simulink library "airlib"  (Simulink 8.7)
settings: Solver=VariableStepAuto  SolverMode=SingleTasking  StartTime=0.0  StopTime=10.0  RelTol=1e-3
undefined symbols (not defined in the file or in its folder): DiscIntNeverNeededParam
libraries: airlib x2
(part 2 of 2)

== system airlib/DT-B747/ad/ad3 ==
  x : Inport
  yatm : Inport  Port=2
  yad1 : Inport  Port=3
  0 : Subsystem
      mask Display: disp('AIRDATA3\nM.O. Rauw, October 1997')
  Mux : Mux  Inputs=3
  Mux1 : Mux  Inputs=[12 5 3]
  Re : Fcn  Expr=(u[13]*u[1])/u[16]
  Tt : Fcn  Expr=u[15] * (1+0.2*u[19]^2)
  cbar : Gain  Gain=cbar  SaturateOnIntegerOverflow=on  OutDataTypeStr=Inherit: Same as input  ParamDataTypeStr=Inherit: Same as input
  yad3 : Outport
  wires:
  yad1/1 -> Mux1/3
  yatm/1 -> Mux1/2
  x/1 -> Mux1/1
  Re/1 -> Mux/2, cbar/1
  Mux1/1 -> Re/1, Tt/1
  Mux/1 -> yad3/1
  Tt/1 -> Mux/1
  cbar/1 -> Mux/3

== system airlib/DT-B747/ad/atm ==
  x : Inport
  0 : Subsystem
      mask Display: disp('ATMOSPH\nM.O. Rauw, October 1997')
  Mux : Mux  Inputs=2
  Mux1 : Mux  Inputs=[2 1]
  Mux2 : Mux  Inputs=5
  T : Fcn  Expr=288.15 - 0.0065*u[12]
  g : Fcn  Expr=9.80665*(6371020/(6371020+u[12]))^2
  mu : Fcn  Expr=(1.458*10^(-6)*u[2]^1.5)/(u[2]+110.4)
  ps : Fcn  Expr=101325*(u[2]/288.15)^(u[1]/1.86584)
  rho : Fcn  Expr=u[3]/(287.053*u[2])
  yatm : Outport
  wires:
  x/1 -> T/1, g/1
  Mux/1 -> Mux1/1, mu/1, ps/1
  ps/1 -> Mux1/2, Mux2/2
  T/1 -> Mux/2, Mux2/3
  g/1 -> Mux/1, Mux2/5
  rho/1 -> Mux2/1
  Mux1/1 -> rho/1
  Mux2/1 -> yatm/1
  mu/1 -> Mux2/4

== system airlib/DT-B747/ae/0 ==

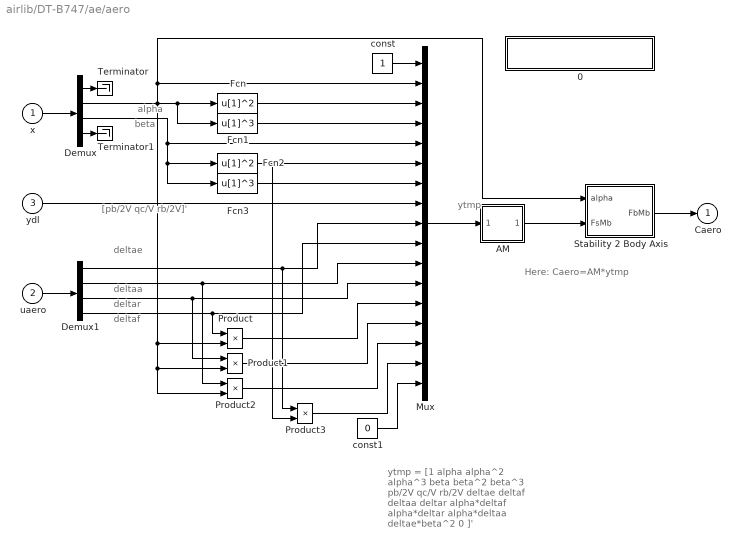
== system airlib/DT-B747/ae/aero ==
  note: ytmp = [1  alpha  alpha^2  alpha^3  beta  beta^2  beta^3  pb/2V  qc/V  rb/2V  deltae
      | deltaf  deltaa  deltar  alpha*deltaf  alpha*deltar  alpha*deltaa  deltae*beta^2  0 ]'
  note: [pb/2V qc/V rb/2V]'
  note: beta
  note: deltae
  note: deltaa
  note: deltar
  note: deltaf
  note: alpha
  note: ytmp
  note: Here: Caero=AM*ytmp
  x : Inport
  uaero : Inport  Port=2
  ydl : Inport  Port=3
  0 : Subsystem
      mask Display: disp('AEROMOD\nM.O. Rauw, October 1997')
  "AM " : Subsystem  mask(State Space){M=AM}
      mask prompts: M "Matrix"
      mask Display: disp('Matrix\nGain')
  Demux : Demux  Outputs=[1 1 1 9]
  Demux1 : Demux
  Fcn : Fcn  Expr=u[1]^2
  Fcn1 : Fcn  Expr=u[1]^3
  Fcn2 : Fcn  Expr=u[1]^2
  Fcn3 : Fcn  Expr=u[1]^3
  Mux : Mux  Inputs=[1 1 1 1 1 1 1 3 1 1 1 1 1 1 1 1 1]
  Product{,1..3} (4 alike) : Product  SaturateOnIntegerOverflow=on  RndMeth=Zero  InputSameDT=on  OutDataTypeStr=Inherit: Same as first input
  Stability 2 Body Axis : Subsystem
  Terminator : Terminator
  Terminator1 : Terminator
  const : Constant
  const1 : Constant  Value=0
  Caero : Outport
  wires:
  Demux/4 -> Terminator1/1
  Demux/1 -> Terminator/1
  const1/1 -> Mux/17
  const/1 -> Mux/1
  ydl/1 -> Mux/8
  Product3/1 -> Mux/16
  Product2/1 -> Mux/15
  Product1/1 -> Mux/14
  Demux1/1 -> Mux/9, Product3/1
  Fcn2/1 -> Mux/6, Product3/2
  Demux1/4 -> Mux/10, Product/1
  Demux/2 -> Fcn/1, Fcn1/1, Product/2, Product1/2, Product2/2, Mux/2, Stability 2 Body Axis/1(alpha)
  Demux/3 -> Mux/5, Fcn2/1, Fcn3/1
  Demux1/2 -> Mux/11, Product2/1
  Demux1/3 -> Mux/12, Product1/1
  Product/1 -> Mux/13
  Fcn3/1 -> Mux/7
  uaero/1 -> Demux1/1
  Fcn1/1 -> Mux/4
  Fcn/1 -> Mux/3
  x/1 -> Demux/1
  Mux/1 -> "AM "/1(In1)
  Stability 2 Body Axis/1(FbMb) -> Caero/1
  "AM "/1(Out1) -> Stability 2 Body Axis/2(FsMb)

== system airlib/DT-B747/ae/dl ==
  x : Inport
  0 : Subsystem
      mask Display: disp('DIMLESS\nM.O. Rauw, October 1997')
  Mux : Mux  Inputs=3
  pb/2V : Fcn  Expr=0.5 * u[4] * b / u[1]
  qc/2V : Fcn  Expr=0.5* u[5] * cbar / u[1]
  rb/2V : Fcn  Expr=0.5 * u[6] * b / u[1]
  ydl : Outport
  wires:
  pb/2V/1 -> Mux/1
  qc/2V/1 -> Mux/2
  rb/2V/1 -> Mux/3
  Mux/1 -> ydl/1
  x/1 -> qc/2V/1, rb/2V/1, pb/2V/1

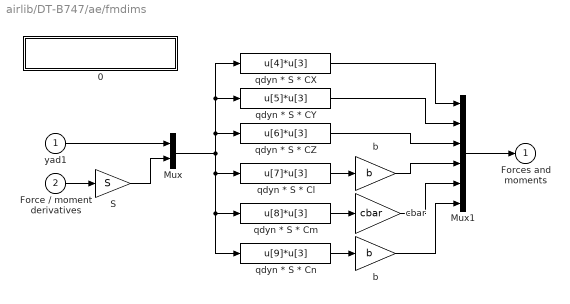
== system airlib/DT-B747/ae/fmdims ==
  yad1 : Inport
  Force / moment derivatives : Inport  Port=2
  0 : Subsystem
      mask Display: disp('FMDIMS\nM.O. Rauw, October 1997')
  Mux : Mux  Inputs=[3 6]
  Mux1 : Mux  Inputs=6
  S : Gain  Gain=S  SaturateOnIntegerOverflow=on  OutDataTypeStr=Inherit: Same as input  ParamDataTypeStr=Inherit: Same as input
  b : Gain  Gain=b  SaturateOnIntegerOverflow=on  OutDataTypeStr=Inherit: Same as input  ParamDataTypeStr=Inherit: Same as input
  "b " : Gain  Gain=b  SaturateOnIntegerOverflow=on  OutDataTypeStr=Inherit: Same as input  ParamDataTypeStr=Inherit: Same as input
  cbar : Gain  Gain=cbar  SaturateOnIntegerOverflow=on  OutDataTypeStr=Inherit: Same as input  ParamDataTypeStr=Inherit: Same as input
  qdyn * S * CX : Fcn  Expr=u[4]*u[3]
  qdyn * S * CY : Fcn  Expr=u[5]*u[3]
  qdyn * S * CZ : Fcn  Expr=u[6]*u[3]
  qdyn * S * Cl : Fcn  Expr=u[7]*u[3]
  qdyn * S * Cm : Fcn  Expr=u[8]*u[3]
  qdyn * S * Cn : Fcn  Expr=u[9]*u[3]
  Forces and moments : Outport
  wires:
  Mux1/1 -> Forces and moments/1
  "b "/1 -> Mux1/6
  cbar/1 -> Mux1/5
  Force / moment derivatives/1 -> S/1
  Mux/1 -> qdyn * S * CZ/1, qdyn * S * CX/1, qdyn * S * CY/1, qdyn * S * Cl/1, qdyn * S * Cm/1, qdyn * S * Cn/1
  qdyn * S * Cl/1 -> b/1
  qdyn * S * Cm/1 -> cbar/1
  qdyn * S * Cn/1 -> "b "/1
  yad1/1 -> Mux/1
  qdyn * S * CX/1 -> Mux1/1
  qdyn * S * CY/1 -> Mux1/2
  S/1 -> Mux/2
  qdyn * S * CZ/1 -> Mux1/3
  b/1 -> Mux1/4

== system airlib/DT-B747/eqm/0 ==

== system airlib/DT-B747/eqm/? ==

== system airlib/DT-B747/eqm/ODE ==
  x : Inport
  Ftot : Inport  Port=2
  Mtot : Inport  Port=3
  yhlp : Inport  Port=4
  ybvel* : Inport  Port=5
  0 : Subsystem
      mask Display: disp('12 Ordinary Differential\nEquations (level 4)\nM.O. Rauw')
  Eulerdot : Subsystem  mask(Eulerdot){}
      mask help:
      | Calculation of d(psi)/dt, d(theta)/dt,
      | and d(phi/dt)
      mask Display: disp('psi dot\ntheta dot\nphi dot')
  Mux : Mux  Inputs=[12 3 3 11]
  Mux1 : Mux  Inputs=[3 3 3 3]
  Vabdot : Subsystem  mask(Vabdot){m=GM1(10)}
      mask prompts: m "Mass of the aircraft [kg]:"
      mask help: Calculation of dV/dt, dalpha/dt, dbeta/dt.
      mask Display: disp('V dot\nalpha dot\nbeta dot')
  pqrdot : Subsystem  mask(pqrdot){}
      mask help: Calculation of dp/dt, dq/dt, and dr/dt
      mask Display: disp('p dot\nq dot\nr dot')
  xyHdot : Subsystem  mask(xyHdot){}
      mask help: Calculation of d(xe)/dt, d(ye)/dt, and dH/dt
      mask Display: disp('xe dot\nye dot\nH dot')
  xdot : Outport
  wires:
  x/1 -> Mux/1
  Mtot/1 -> Mux/3
  Ftot/1 -> Mux/2
  Mux/1 -> pqrdot/1(upqr), Vabdot/1(uVab), Eulerdot/1(ueul), xyHdot/2(uxYH)
  ybvel*/1 -> xyHdot/1(ybvel*)
  yhlp/1 -> Mux/4
  xyHdot/1(yxyH) -> Mux1/4
  Eulerdot/1(yeul) -> Mux1/3
  pqrdot/1(ypqr) -> Mux1/2
  Vabdot/1(yVab) -> Mux1/1
  Mux1/1 -> xdot/1

== system airlib/DT-B747/eqm/uvw ==
  yhlp : Inport
  x : Inport  Port=2
  0 : Subsystem
      mask Display: disp('UVW\nM.O. Rauw, October 1997')
  Mux : Mux  Inputs=3
  Mux1 : Mux  Inputs=[12 11]
  u : Fcn  Expr=u[1]*u[13]*u[15]
  v : Fcn  Expr=u[1]*u[16]
  w : Fcn  Expr=u[1]*u[14]*u[15]
  ybvel : Outport
  wires:
  Mux1/1 -> v/1, u/1, w/1
  yhlp/1 -> Mux1/2
  x/1 -> Mux1/1
  u/1 -> Mux/1
  v/1 -> Mux/2
  w/1 -> Mux/3
  Mux/1 -> ybvel/1

== system airlib/DT-B747/eqm/xdotcorr ==
  xdot uncorrected : Inport
  yhlp : Inport  Port=2
  yatm : Inport  Port=3
  0 : Subsystem
      mask Display: disp('XDOTCORR (General)\nM.O. Rauw, October 1997')
  Demux : Demux  Outputs=12
  Mux1 : Mux  Inputs=12
  Mux2 : Mux  Inputs=[11 1 5]
  beta dot correction : Fcn  Expr=u[12] / (1 - (u[3]*u[13]*b*S*CYbdot)/(4*m))
  xdot corrected : Outport
  wires:
  beta dot correction/1 -> Mux1/3
  yatm/1 -> Mux2/3
  Demux/1 -> Mux1/1
  Demux/2 -> Mux1/2
  Demux/4 -> Mux1/4
  Demux/5 -> Mux1/5
  Demux/6 -> Mux1/6
  Demux/7 -> Mux1/7
  Demux/8 -> Mux1/8
  Demux/9 -> Mux1/9
  Demux/10 -> Mux1/10
  Demux/11 -> Mux1/11
  Demux/12 -> Mux1/12
  Demux/3 -> Mux2/2
  xdot uncorrected/1 -> Demux/1
  Mux1/1 -> xdot corrected/1
  Mux2/1 -> beta dot correction/1
  yhlp/1 -> Mux2/1

== system airlib/DT-B747/fms/0 ==

== system airlib/DT-B747/fw/0 ==

== system airlib/DT-B747/gr/0 ==

== system airlib/DT-B747/hlp/0 ==

== system airlib/DT-B747/out/0 ==

== system airlib/DT-B747/out/accel ==
  Ftot : Inport
  Fgrav : Inport  Port=2
  0 : Subsystem
      mask Display: disp('ACCEL\nM.O. Rauw, October 1997')
  Ax : Fcn  Expr=(u[1]-u[4])/(m*9.80665)
  Ay : Fcn  Expr=(u[2]-u[5])/(m*9.80665)
  Az : Fcn  Expr=(u[3]-u[6])/(m*9.80665)
  Mux : Mux  Inputs=6
  Mux1 : Mux  Inputs=[3 3]
  axk : Fcn  Expr=u[1]/(m*9.80665)
  ayk : Fcn  Expr=u[2]/(m*9.80665)
  azk : Fcn  Expr=u[3]/(m*9.80665)
  yacc : Outport
  wires:
  Ftot/1 -> Mux1/1
  Fgrav/1 -> Mux1/2
  Mux/1 -> yacc/1
  azk/1 -> Mux/6
  Az/1 -> Mux/3
  Ay/1 -> Mux/2
  Ax/1 -> Mux/1
  Mux1/1 -> Az/1, Ax/1, Ay/1, axk/1, azk/1, ayk/1
  axk/1 -> Mux/4
  ayk/1 -> Mux/5

== system airlib/DT-B747/out/fp ==
  x : Inport
  xdot : Inport  Port=2
  0 : Subsystem
      mask Display: disp('FLPATH\nM.O. Rauw, October 1997')
  Mux : Mux  Inputs=[12 12]
  Mux1 : Mux
  Phi : Fcn  Expr=u[9]*cos(u[8]-alpha0)
  chi : Fcn  Expr=u[3]+u[7]
  fpa : Fcn  Expr=u[13]/9.80665
  gamma : Fcn  Expr=asin(u[24]/u[1])
  yfp : Outport
  wires:
  gamma/1 -> Mux1/1
  Mux/1 -> chi/1, Phi/1, fpa/1, gamma/1
  fpa/1 -> Mux1/2
  chi/1 -> Mux1/3
  Phi/1 -> Mux1/4
  Mux1/1 -> yfp/1
  x/1 -> Mux/1
  xdot/1 -> Mux/2

== system airlib/DT-B747/out/uvwdot ==
  note: `
  note: cos(alpha)
  note: sin(alpha)
  note: cos(beta)
  note: sin(beta)
  note: V
  x : Inport
  xdot : Inport  Port=2
  yhlp : Inport  Port=3
  0 : Subsystem
      mask Display: disp('UVWDOT\nM.O. Rauw, October 1997')
  DeMux : Demux  Outputs=[1 1 1 1 7]
  Demux : Demux  Outputs=[1 11]
  Mux : Mux  Inputs=[1 1 1 1 1 12]
  Mux1 : Mux  Inputs=3
  Terminator : Terminator
  Terminator1 : Terminator
  u dot : Fcn  Expr=u[6]*u[1]*u[3] - u[5]*(u[7]*u[2]*u[3] + u[8]*u[1]*u[4])
  v dot : Fcn  Expr=u[6]*u[4] + u[5]*u[3]*u[8]
  wdot : Fcn  Expr=u[6]*u[2]*u[3] + u[5]*(u[7]*u[1]*u[3] - u[8]*u[2]*u[4])
  yuvw =  [udot; vdot; wdot] : Outport
  wires:
  Demux/2 -> Terminator1/1
  DeMux/5 -> Terminator/1
  wdot/1 -> Mux1/3
  v dot/1 -> Mux1/2
  u dot/1 -> Mux1/1
  xdot/1 -> Mux/6
  Mux/1 -> v dot/1, wdot/1, u dot/1
  DeMux/1 -> Mux/1
  DeMux/2 -> Mux/2
  x/1 -> Demux/1
  Mux1/1 -> yuvw =  [udot; vdot; wdot]/1
  yhlp/1 -> DeMux/1
  DeMux/3 -> Mux/3
  DeMux/4 -> Mux/4
  Demux/1 -> Mux/5

== system airlib/B747/ad/ad1/0 ==

== system airlib/B747/ad/ad2/0 ==

== system airlib/B747/ad/ad3/0 ==

== system airlib/B747/ad/atm/0 ==

== system airlib/B747/ae/aero/0 ==

== system airlib/B747/ae/aero/AM  ==
  In1 : Inport
  Display : Display
  Display1 : Display
  Matrix Gain : StateSpace  A=[]  B=[]  C=[]  D=M  X0=0
  Out1 : Outport
  wires:
  Matrix Gain/1 -> Out1/1, Display/1
  In1/1 -> Matrix Gain/1, Display1/1

== system airlib/B747/ae/aero/Stability 2 Body Axis ==
  alpha : Inport
  FsMb : Inport  Port=2
  Demux2 : Demux  Outputs=6
  Mux1 : Mux  Inputs=6
  Product{2..5} (4 alike) : Product  SaturateOnIntegerOverflow=on  RndMeth=Zero  InputSameDT=on  OutDataTypeStr=Inherit: Same as first input
  Sum3 : Sum  Inputs=-+  SaturateOnIntegerOverflow=on  InputSameDT=on  OutDataTypeStr=Inherit: Same as first input
  Sum4 : Sum  Inputs=--  SaturateOnIntegerOverflow=on  InputSameDT=on  OutDataTypeStr=Inherit: Same as first input
  cos alpha : Fcn  Expr=cos(u[1])
  sin alpha : Fcn
  FbMb : Outport
  wires:
  FsMb/1 -> Demux2/1
  Mux1/1 -> FbMb/1
  alpha/1 -> cos alpha/1, sin alpha/1
  Sum4/1 -> Mux1/3
  Product5/1 -> Sum4/2
  Product4/1 -> Sum4/1
  Demux2/3 -> Product5/2, Product3/2
  sin alpha/1 -> Product4/1, Product3/1
  Sum3/1 -> Mux1/1
  Product3/1 -> Sum3/2
  Product2/1 -> Sum3/1
  Demux2/1 -> Product4/2, Product2/2
  cos alpha/1 -> Product5/1, Product2/1
  Demux2/4 -> Mux1/4
  Demux2/2 -> Mux1/2
  Demux2/5 -> Mux1/5
  Demux2/6 -> Mux1/6

== system airlib/B747/ae/dl/0 ==

== system airlib/B747/ae/fmdims/0 ==

== system airlib/B747/eqm/ODE/0 ==

== system airlib/B747/eqm/ODE/Eulerdot ==
  note: yeul=[psi dot; theta dot; phi dot]
  note: ueul=[x;Ftot;Mtot;yhlp]
  ueul : Inport
  0 : Subsystem
      mask Display: disp('EULERDOT\nM.O. Rauw, October 1997')
  Mux1 : Mux  Inputs=[29 1]
  Mux2 : Mux  Inputs=3
  phi dot : Fcn  Expr=u[4] + u[30]*u[26]
  psi dot : Fcn  Expr=(u[5]*u[28] + u[6]*u[29])/u[27]
  theta dot : Fcn  Expr=u[5]*u[29] - u[6]*u[28]
  yeul : Outport
  wires:
  Mux1/1 -> phi dot/1
  phi dot/1 -> Mux2/3
  Mux2/1 -> yeul/1
  theta dot/1 -> Mux2/2
  psi dot/1 -> Mux1/2, Mux2/1
  ueul/1 -> psi dot/1, Mux1/1, theta dot/1

== system airlib/B747/eqm/ODE/Vabdot ==
  note: uVab=[x;Ftot;Mtot;yhlp]
  note: yVab=[V dot;alpha dot;beta dot]
  uVab : Inport
  0 : Subsystem
      mask Display: disp('VABDOT\nM.O. Rauw, October 1997')
  Mux2 : Mux  Inputs=3
  V dot : Fcn  Expr=(u[13]*u[19]*u[21]+u[14]*u[22]+u[15]*u[20]*u[21])/m
  alpha dot : Fcn  Expr=(-u[13]*u[20]+u[15]*u[19])/(m*u[1]*u[21]) - u[23]*(u[4]*u[19]+u[6]*u[20]) + u[5]
  beta dot : Fcn  Expr=(-u[13]*u[19]*u[22]+u[14]*u[21]-u[15]*u[20]*u[22])/(m*u[1]) + u[4]*u[20] - u[6]*u[19]
  yVab : Outport
  wires:
  Mux2/1 -> yVab/1
  uVab/1 -> V dot/1, beta dot/1, alpha dot/1
  alpha dot/1 -> Mux2/2
  V dot/1 -> Mux2/1
  beta dot/1 -> Mux2/3

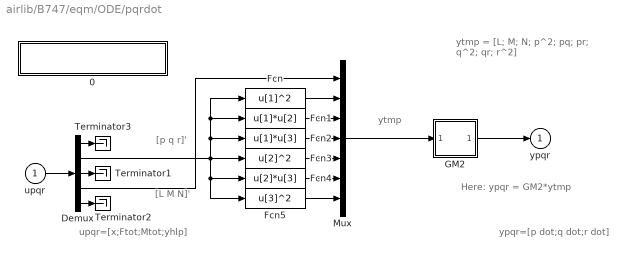
== system airlib/B747/eqm/ODE/pqrdot ==
  note: [p q r]'
  note: [L M N]'
  note: Here: ypqr = GM2*ytmp
  note: ytmp
  note: ypqr=[p dot;q dot;r dot]
  note: upqr=[x;Ftot;Mtot;yhlp]
  note: ytmp = [L; M; N; p^2; pq; pr; q^2; qr; r^2]
  upqr : Inport
  0 : Subsystem
      mask Display: disp('PQRDOT\nM.O. Rauw, October 1997')
  Demux : Demux  Outputs=[3 3 9 3 11]
  Fcn : Fcn  Expr=u[1]^2
  Fcn1 : Fcn  Expr=u[1]*u[2]
  Fcn2 : Fcn  Expr=u[1]*u[3]
  Fcn3 : Fcn  Expr=u[2]^2
  Fcn4 : Fcn  Expr=u[2]*u[3]
  Fcn5 : Fcn  Expr=u[3]^2
  "GM2 " : Subsystem  mask(State Space){M=GM2}
      mask prompts: M "Matrix"
      mask Display: disp('Matrix\nGain')
  Mux : Mux  Inputs=[3 1 1 1 1 1 1]
  Terminator1 : Terminator
  Terminator2 : Terminator
  Terminator3 : Terminator
  ypqr : Outport
  wires:
  upqr/1 -> Demux/1
  Demux/1 -> Terminator3/1
  Demux/5 -> Terminator2/1
  Demux/3 -> Terminator1/1
  Demux/2 -> Fcn1/1, Fcn/1, Fcn2/1, Fcn4/1, Fcn5/1, Fcn3/1
  Demux/4 -> Mux/1
  Fcn/1 -> Mux/2
  Fcn1/1 -> Mux/3
  Fcn2/1 -> Mux/4
  Fcn3/1 -> Mux/5
  Fcn4/1 -> Mux/6
  Fcn5/1 -> Mux/7
  "GM2 "/1(Out1) -> ypqr/1
  Mux/1 -> "GM2 "/1(In1)

== system airlib/B747/eqm/ODE/xyHdot ==
  note: yxyH=[xe dot; ye dot; H dot]
  note: uxyH=[x;Ftot;Mtot;yhlp]
  ybvel* : Inport
  uxYH : Inport  Port=2
  0 : Subsystem
      mask Display: disp('XYHDOT\nM.O. Rauw, October 1997')
  H dot : Fcn  Expr=u[30]*u[26] - (u[31]*u[28]+u[32]*u[29])*u[27]
  Mux2 : Mux  Inputs=[29 3]
  Mux3 : Mux  Inputs=2
  Mux4 : Mux  Inputs=[29 2]
  Mux5 : Mux  Inputs=3
  tmp1 : Fcn  Expr=u[30]*u[27] + (u[31]*u[28]+u[32]*u[29])*u[26]
  tmp2 : Fcn  Expr=u[31]*u[29] - u[32]*u[28]
  xe dot : Fcn  Expr=u[30]*u[25] - u[31]*u[24]
  ye dot : Fcn  Expr=u[30]*u[24] + u[31]*u[25]
  yxyH : Outport
  wires:
  tmp1/1 -> Mux3/1
  H dot/1 -> Mux5/3
  xe dot/1 -> Mux5/1
  tmp2/1 -> Mux3/2
  ye dot/1 -> Mux5/2
  Mux5/1 -> yxyH/1
  Mux4/1 -> ye dot/1, xe dot/1
  Mux2/1 -> H dot/1, tmp2/1, tmp1/1
  Mux3/1 -> Mux4/2
  ybvel*/1 -> Mux2/2
  uxYH/1 -> Mux4/1, Mux2/1

== system airlib/B747/eqm/uvw/0 ==

== system airlib/B747/eqm/xdotcorr/0 ==

== system airlib/B747/out/accel/0 ==

== system airlib/B747/out/fp/0 ==

== system airlib/B747/out/uvwdot/0 ==

== system airlib/DT-B747/ad/ad1/0 ==

== system airlib/DT-B747/ad/ad2/0 ==

== system airlib/DT-B747/ad/ad3/0 ==

== system airlib/DT-B747/ad/atm/0 ==

== system airlib/DT-B747/ae/aero/0 ==

== system airlib/DT-B747/ae/aero/AM  ==
  In1 : Inport
  Matrix Gain : StateSpace  A=[]  B=[]  C=[]  D=M  X0=0
  Out1 : Outport
  wires:
  In1/1 -> Matrix Gain/1
  Matrix Gain/1 -> Out1/1

== system airlib/DT-B747/ae/aero/Stability 2 Body Axis ==
  alpha : Inport
  FsMb : Inport  Port=2
  Demux2 : Demux  Outputs=6
  Mux1 : Mux  Inputs=6
  Product{2..5} (4 alike) : Product  SaturateOnIntegerOverflow=on  RndMeth=Zero  InputSameDT=on  OutDataTypeStr=Inherit: Same as first input
  Sum3 : Sum  Inputs=-+  SaturateOnIntegerOverflow=on  InputSameDT=on  OutDataTypeStr=Inherit: Same as first input
  Sum4 : Sum  Inputs=--  SaturateOnIntegerOverflow=on  InputSameDT=on  OutDataTypeStr=Inherit: Same as first input
  cos alpha : Fcn  Expr=cos(u[1])
  sin alpha : Fcn
  FbMb : Outport
  wires:
  Demux2/6 -> Mux1/6
  Demux2/5 -> Mux1/5
  Demux2/2 -> Mux1/2
  Demux2/4 -> Mux1/4
  cos alpha/1 -> Product2/1, Product5/1
  Demux2/1 -> Product2/2, Product4/2
  Product2/1 -> Sum3/1
  Product3/1 -> Sum3/2
  Sum3/1 -> Mux1/1
  sin alpha/1 -> Product3/1, Product4/1
  Demux2/3 -> Product3/2, Product5/2
  Product4/1 -> Sum4/1
  Product5/1 -> Sum4/2
  Sum4/1 -> Mux1/3
  alpha/1 -> sin alpha/1, cos alpha/1
  Mux1/1 -> FbMb/1
  FsMb/1 -> Demux2/1

== system airlib/DT-B747/ae/dl/0 ==

== system airlib/DT-B747/ae/fmdims/0 ==

== system airlib/DT-B747/eqm/ODE/0 ==

== system airlib/DT-B747/eqm/ODE/Eulerdot ==
  note: ueul=[x;Ftot;Mtot;yhlp]
  note: yeul=[psi dot; theta dot; phi dot]
  ueul : Inport
  0 : Subsystem
      mask Display: disp('EULERDOT\nM.O. Rauw, October 1997')
  Mux1 : Mux  Inputs=[29 1]
  Mux2 : Mux  Inputs=3
  phi dot : Fcn  Expr=u[4] + u[30]*u[26]
  psi dot : Fcn  Expr=(u[5]*u[28] + u[6]*u[29])/u[27]
  theta dot : Fcn  Expr=u[5]*u[29] - u[6]*u[28]
  yeul : Outport
  wires:
  ueul/1 -> theta dot/1, Mux1/1, psi dot/1
  psi dot/1 -> Mux2/1, Mux1/2
  theta dot/1 -> Mux2/2
  Mux2/1 -> yeul/1
  phi dot/1 -> Mux2/3
  Mux1/1 -> phi dot/1

== system airlib/DT-B747/eqm/ODE/Vabdot ==
  note: yVab=[V dot;alpha dot;beta dot]
  note: uVab=[x;Ftot;Mtot;yhlp]
  uVab : Inport
  0 : Subsystem
      mask Display: disp('VABDOT\nM.O. Rauw, October 1997')
  Mux2 : Mux  Inputs=3
  V dot : Fcn  Expr=(u[13]*u[19]*u[21]+u[14]*u[22]+u[15]*u[20]*u[21])/m
  alpha dot : Fcn  Expr=(-u[13]*u[20]+u[15]*u[19])/(m*u[1]*u[21]) - u[23]*(u[4]*u[19]+u[6]*u[20]) + u[5]
  beta dot : Fcn  Expr=(-u[13]*u[19]*u[22]+u[14]*u[21]-u[15]*u[20]*u[22])/(m*u[1]) + u[4]*u[20] - u[6]*u[19]
  yVab : Outport
  wires:
  beta dot/1 -> Mux2/3
  V dot/1 -> Mux2/1
  alpha dot/1 -> Mux2/2
  uVab/1 -> alpha dot/1, beta dot/1, V dot/1
  Mux2/1 -> yVab/1

== system airlib/DT-B747/eqm/ODE/pqrdot ==
  note: ytmp = [L; M; N; p^2; pq; pr; q^2; qr; r^2]
  note: upqr=[x;Ftot;Mtot;yhlp]
  note: ypqr=[p dot;q dot;r dot]
  note: ytmp
  note: Here: ypqr = GM2*ytmp
  note: [L M N]'
  note: [p q r]'
  upqr : Inport
  0 : Subsystem
      mask Display: disp('PQRDOT\nM.O. Rauw, October 1997')
  Demux : Demux  Outputs=[3 3 9 3 11]
  Fcn : Fcn  Expr=u[1]^2
  Fcn1 : Fcn  Expr=u[1]*u[2]
  Fcn2 : Fcn  Expr=u[1]*u[3]
  Fcn3 : Fcn  Expr=u[2]^2
  Fcn4 : Fcn  Expr=u[2]*u[3]
  Fcn5 : Fcn  Expr=u[3]^2
  "GM2 " : Subsystem  mask(State Space){M=GM2}
      mask prompts: M "Matrix"
      mask Display: disp('Matrix\nGain')
  Mux : Mux  Inputs=[3 1 1 1 1 1 1]
  Terminator1 : Terminator
  Terminator2 : Terminator
  Terminator3 : Terminator
  ypqr : Outport
  wires:
  Mux/1 -> "GM2 "/1(In1)
  "GM2 "/1(Out1) -> ypqr/1
  Fcn5/1 -> Mux/7
  Fcn4/1 -> Mux/6
  Fcn3/1 -> Mux/5
  Fcn2/1 -> Mux/4
  Fcn1/1 -> Mux/3
  Fcn/1 -> Mux/2
  Demux/4 -> Mux/1
  Demux/2 -> Fcn3/1, Fcn5/1, Fcn4/1, Fcn2/1, Fcn/1, Fcn1/1
  Demux/3 -> Terminator1/1
  Demux/5 -> Terminator2/1
  Demux/1 -> Terminator3/1
  upqr/1 -> Demux/1

== system airlib/DT-B747/eqm/ODE/xyHdot ==
  note: uxyH=[x;Ftot;Mtot;yhlp]
  note: yxyH=[xe dot; ye dot; H dot]
  ybvel* : Inport
  uxYH : Inport  Port=2
  0 : Subsystem
      mask Display: disp('XYHDOT\nM.O. Rauw, October 1997')
  H dot : Fcn  Expr=u[30]*u[26] - (u[31]*u[28]+u[32]*u[29])*u[27]
  Mux2 : Mux  Inputs=[29 3]
  Mux3 : Mux  Inputs=2
  Mux4 : Mux  Inputs=[29 2]
  Mux5 : Mux  Inputs=3
  tmp1 : Fcn  Expr=u[30]*u[27] + (u[31]*u[28]+u[32]*u[29])*u[26]
  tmp2 : Fcn  Expr=u[31]*u[29] - u[32]*u[28]
  xe dot : Fcn  Expr=u[30]*u[25] - u[31]*u[24]
  ye dot : Fcn  Expr=u[30]*u[24] + u[31]*u[25]
  yxyH : Outport
  wires:
  uxYH/1 -> Mux2/1, Mux4/1
  ybvel*/1 -> Mux2/2
  Mux3/1 -> Mux4/2
  Mux2/1 -> tmp1/1, tmp2/1, H dot/1
  Mux4/1 -> xe dot/1, ye dot/1
  Mux5/1 -> yxyH/1
  ye dot/1 -> Mux5/2
  tmp2/1 -> Mux3/2
  xe dot/1 -> Mux5/1
  H dot/1 -> Mux5/3
  tmp1/1 -> Mux3/1

== system airlib/DT-B747/eqm/uvw/0 ==

== system airlib/DT-B747/eqm/xdotcorr/0 ==

== system airlib/DT-B747/out/accel/0 ==

== system airlib/DT-B747/out/fp/0 ==

== system airlib/DT-B747/out/uvwdot/0 ==

== system airlib/B747/eqm/ODE/Eulerdot/0 ==

== system airlib/B747/eqm/ODE/Vabdot/0 ==

== system airlib/B747/eqm/ODE/pqrdot/0 ==

== system airlib/B747/eqm/ODE/pqrdot/GM2  ==
  In1 : Inport
  Matrix Gain : StateSpace  A=[]  B=[]  C=[]  D=M  X0=0
  Out1 : Outport
  wires:
  Matrix Gain/1 -> Out1/1
  In1/1 -> Matrix Gain/1

== system airlib/B747/eqm/ODE/xyHdot/0 ==

== system airlib/DT-B747/eqm/ODE/Eulerdot/0 ==

== system airlib/DT-B747/eqm/ODE/Vabdot/0 ==

== system airlib/DT-B747/eqm/ODE/pqrdot/0 ==

== system airlib/DT-B747/eqm/ODE/pqrdot/GM2  ==
  In1 : Inport
  Matrix Gain : StateSpace  A=[]  B=[]  C=[]  D=M  X0=0
  Out1 : Outport
  wires:
  In1/1 -> Matrix Gain/1
  Matrix Gain/1 -> Out1/1

== system airlib/DT-B747/eqm/ODE/xyHdot/0 ==
